simulink model "Incremental_HSMC"  (R2023b)
settings: Solver=ode1  StartTime=0.0  StopTime=60  FixedStep=0.01  RelTol=1e-3
libraries: simulink x1
settings Model: Creator=vanch  LastModifiedBy=vanch

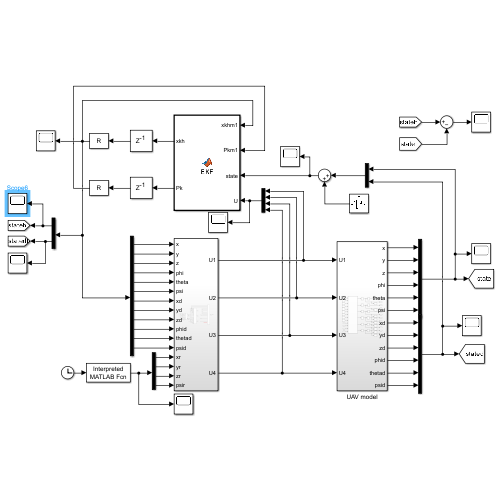
[thumbnail: Simulink's stored preview of the top-level diagram]
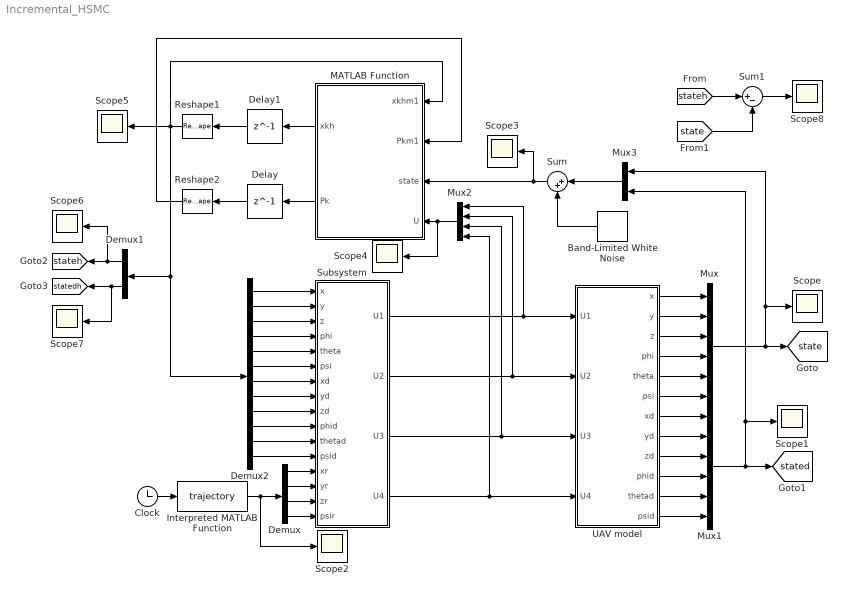
== system Incremental_HSMC ==
  Band-Limited White Noise : simulink/Sources/Band-Limited White Noise  Cov=1e-8  Ts=0.01  seed=[1535]
  Clock : Clock
  Delay : Delay  DelayLength=1  InitialCondition=(1e-3)*eye(12,12)
  Delay1 : Delay  DelayLength=1  InitialCondition=0.001
  Demux : Demux
  Demux1 : Demux  Outputs=2
  Demux2 : Demux  Outputs=12
  Interpreted MATLAB Function : MATLABFcn  MATLABFcn=trajectory  OutputDimensions=4
  MATLAB Function : MATLAB Function  TreatAsAtomicUnit=on
  Mux : Mux  Inputs=6
  Mux1 : Mux  Inputs=6
  Mux2 : Mux
  Mux3 : Mux  Inputs=2
  Reshape1 : Reshape  OutputDimensionality=Customize  OutputDimensions=[12,1]
  Reshape2 : Reshape  OutputDimensionality=Customize  OutputDimensions=[12,12]
  Scope{,1..8} (9 alike) : Scope
  Subsystem : Subsystem
  Sum : Sum  Inputs=|++
  Sum1 : Sum  Inputs=|+-
  UAV model : Subsystem
  tag scope: state=global, stated=global, statedh=global, stateh=global
  wires:
  UAV model/1(x) -> Mux/1
  UAV model/2(y) -> Mux/2
  UAV model/3(z) -> Mux/3
  UAV model/4(phi) -> Mux/4
  UAV model/5(theta) -> Mux/5
  UAV model/6(psi) -> Mux/6
  UAV model/7(xd) -> Mux1/1
  UAV model/8(yd) -> Mux1/2
  UAV model/9(zd) -> Mux1/3
  UAV model/10(phid) -> Mux1/4
  UAV model/11(thetad) -> Mux1/5
  UAV model/12(psid) -> Mux1/6
  Subsystem/3(U3) -> UAV model/3(U3), Mux2/3
  Subsystem/1(U1) -> Mux2/1, UAV model/1(U1)
  Mux/1 -> [state], Scope/1, Mux3/1
  Subsystem/4(U4) -> Mux2/4, UAV model/4(U4)
  Mux3/1 -> Sum/1
  Mux1/1 -> Mux3/2, Scope1/1, [stated]
  Subsystem/2(U2) -> Mux2/2, UAV model/2(U2)
  Mux2/1 -> Scope4/1, MATLAB Function/4(U)
  MATLAB Function/1(xkh) -> Delay1/1
  MATLAB Function/2(Pk) -> Delay/1
  Delay/1 -> Reshape2/1
  Reshape2/1 -> MATLAB Function/2(Pkm1)
  Sum/1 -> MATLAB Function/3(state), Scope3/1
  Delay1/1 -> Reshape1/1
  Demux2/4 -> Subsystem/4(phi)
  Demux2/5 -> Subsystem/5(theta)
  Demux2/6 -> Subsystem/6(psi)
  Demux2/7 -> Subsystem/7(xd)
  Demux2/8 -> Subsystem/8(yd)
  Demux2/9 -> Subsystem/9(zd)
  Demux2/10 -> Subsystem/10(phid)
  Demux2/11 -> Subsystem/11(thetad)
  Demux2/12 -> Subsystem/12(psid)
  Demux2/1 -> Subsystem/1(x)
  Demux2/2 -> Subsystem/2(y)
  Demux2/3 -> Subsystem/3(z)
  Clock/1 -> Interpreted MATLAB Function/1
  Demux/2 -> Subsystem/14(yr)
  Demux/4 -> Subsystem/16(psir)
  Demux/3 -> Subsystem/15(zr)
  Demux/1 -> Subsystem/13(xr)
  Interpreted MATLAB Function/1 -> Demux/1, Scope2/1
  Demux1/2 -> Scope7/1, [statedh]
  Reshape1/1 -> MATLAB Function/1(xkhm1), Demux2/1, Demux1/1, Scope5/1
  Demux1/1 -> Scope6/1, [stateh]
  Sum1/1 -> Scope8/1
  [stateh] -> Sum1/1
  [state] -> Sum1/2
  Band-Limited White Noise/1 -> Sum/2

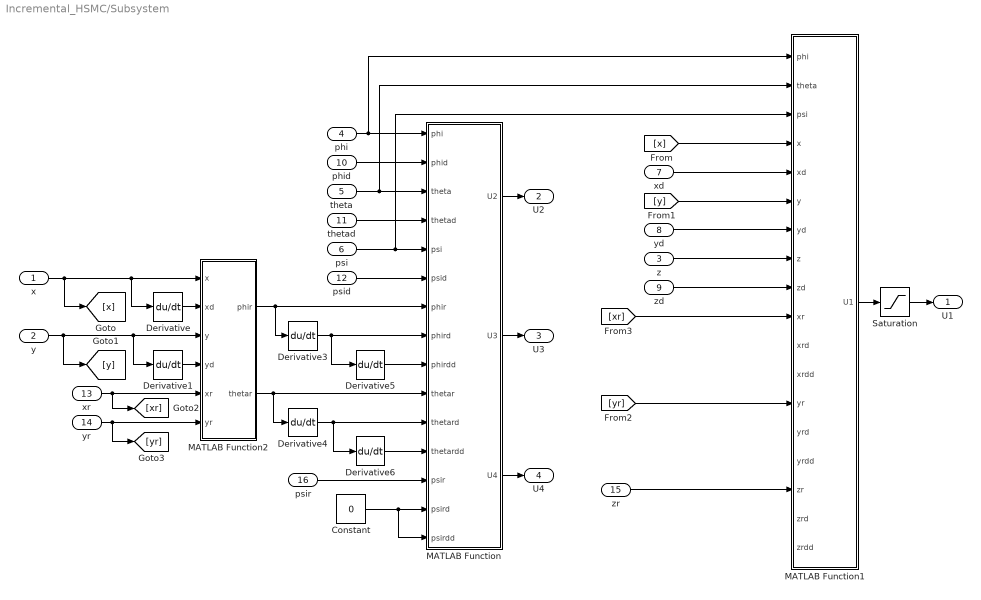
== system Incremental_HSMC/Subsystem ==
  x : Inport
  y : Inport  Port=2
  z : Inport  Port=3
  phi : Inport  Port=4
  theta : Inport  Port=5
  psi : Inport  Port=6
  xd : Inport  Port=7
  yd : Inport  Port=8
  zd : Inport  Port=9
  phid : Inport  Port=10
  thetad : Inport  Port=11
  psid : Inport  Port=12
  xr : Inport  Port=13
  yr : Inport  Port=14
  zr : Inport  Port=15
  psir : Inport  Port=16
  Constant : Constant  Value=0
  Derivative{,1,3..6} (6 alike) : Derivative
  MATLAB Function : MATLAB Function  TreatAsAtomicUnit=on
  MATLAB Function1 : MATLAB Function  TreatAsAtomicUnit=on
  MATLAB Function2 : MATLAB Function  TreatAsAtomicUnit=on
  Saturation : Saturate  UpperLimit=50  LowerLimit=0
  U1 : Outport
  U2 : Outport  Port=2
  U3 : Outport  Port=3
  U4 : Outport  Port=4
  wires:
  x/1 -> Derivative/1, MATLAB Function2/1(x), [x]
  Derivative/1 -> MATLAB Function2/2(xd)
  Derivative1/1 -> MATLAB Function2/4(yd)
  y/1 -> [y], Derivative1/1, MATLAB Function2/3(y)
  xr/1 -> [xr], MATLAB Function2/5(xr)
  yr/1 -> [yr], MATLAB Function2/6(yr)
  MATLAB Function/1(U2) -> U2/1
  MATLAB Function/2(U3) -> U3/1
  MATLAB Function/3(U4) -> U4/1
  phi/1 -> MATLAB Function/1(phi), MATLAB Function1/1(phi)
  theta/1 -> MATLAB Function/3(theta), MATLAB Function1/2(theta)
  psi/1 -> MATLAB Function/5(psi), MATLAB Function1/3(psi)
  MATLAB Function2/1(phir) -> MATLAB Function/7(phir), Derivative3/1
  MATLAB Function2/2(thetar) -> MATLAB Function/10(thetar), Derivative4/1
  phid/1 -> MATLAB Function/2(phid)
  thetad/1 -> MATLAB Function/4(thetad)
  Derivative3/1 -> Derivative5/1, MATLAB Function/8(phird)
  Derivative4/1 -> Derivative6/1, MATLAB Function/11(thetard)
  psid/1 -> MATLAB Function/6(psid)
  psir/1 -> MATLAB Function/13(psir)
  Derivative5/1 -> MATLAB Function/9(phirdd)
  Derivative6/1 -> MATLAB Function/12(thetardd)
  [x] -> MATLAB Function1/4(x)
  [y] -> MATLAB Function1/6(y)
  xd/1 -> MATLAB Function1/5(xd)
  yd/1 -> MATLAB Function1/7(yd)
  z/1 -> MATLAB Function1/8(z)
  zd/1 -> MATLAB Function1/9(zd)
  zr/1 -> MATLAB Function1/16(zr)
  ? -> MATLAB Function1/17(zrd)
  [yr] -> MATLAB Function1/13(yr)
  [xr] -> MATLAB Function1/10(xr)
  Constant/1 -> MATLAB Function/15(psirdd), MATLAB Function/14(psird)
  MATLAB Function1/1(U1) -> Saturation/1
  Saturation/1 -> U1/1

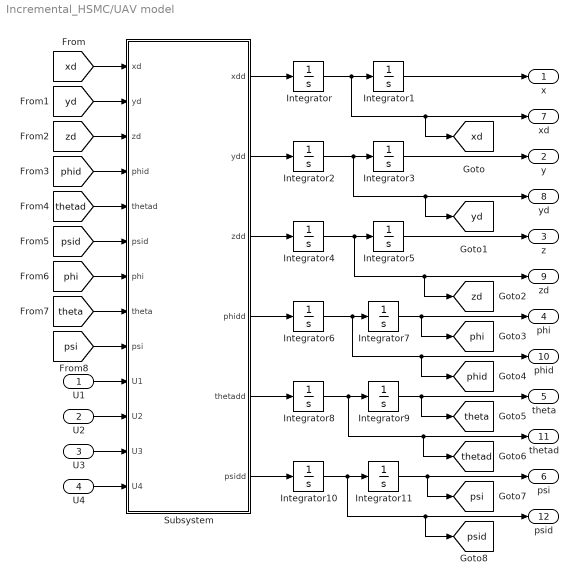
== system Incremental_HSMC/UAV model ==
  U1 : Inport
  U2 : Inport  Port=2
  U3 : Inport  Port=3
  U4 : Inport  Port=4
  Integrator{,1,3,7,9,11} (6 alike) : Integrator  InitialCondition=0.01
  Integrator{2,4,6,8,10} (5 alike) : Integrator
  Integrator5 : Integrator  InitialCondition=0.01  LimitOutput=on  LowerSaturationLimit=0
  Subsystem : Subsystem
  x : Outport
  y : Outport  Port=2
  z : Outport  Port=3
  phi : Outport  Port=4
  theta : Outport  Port=5
  psi : Outport  Port=6
  xd : Outport  Port=7
  yd : Outport  Port=8
  zd : Outport  Port=9
  phid : Outport  Port=10
  thetad : Outport  Port=11
  psid : Outport  Port=12
  tag scope: phi=global, phid=global, psi=global, psid=global, theta=global, thetad=global, xd=global, yd=global, zd=global
  wires:
  Integrator5/1 -> z/1
  Integrator6/1 -> phid/1, [phid], Integrator7/1
  Integrator1/1 -> x/1
  [psid] -> Subsystem/6(psid)
  Integrator2/1 -> yd/1, [yd], Integrator3/1
  Subsystem/3(zdd) -> Integrator4/1
  Subsystem/6(psidd) -> Integrator10/1
  Integrator3/1 -> y/1
  Integrator8/1 -> thetad/1, [thetad], Integrator9/1
  [theta] -> Subsystem/8(theta)
  Integrator/1 -> xd/1, [xd], Integrator1/1
  [thetad] -> Subsystem/5(thetad)
  [zd] -> Subsystem/3(zd)
  Subsystem/4(phidd) -> Integrator6/1
  Integrator9/1 -> theta/1, [theta]
  [phid] -> Subsystem/4(phid)
  Integrator10/1 -> psid/1, [psid], Integrator11/1
  Subsystem/2(ydd) -> Integrator2/1
  Integrator4/1 -> zd/1, [zd], Integrator5/1
  Subsystem/5(thetadd) -> Integrator8/1
  Subsystem/1(xdd) -> Integrator/1
  [yd] -> Subsystem/2(yd)
  [psi] -> Subsystem/9(psi)
  Integrator11/1 -> psi/1, [psi]
  [xd] -> Subsystem/1(xd)
  [phi] -> Subsystem/7(phi)
  Integrator7/1 -> phi/1, [phi]
  U1/1 -> Subsystem/10(U1)
  U2/1 -> Subsystem/11(U2)
  U3/1 -> Subsystem/12(U3)
  U4/1 -> Subsystem/13(U4)

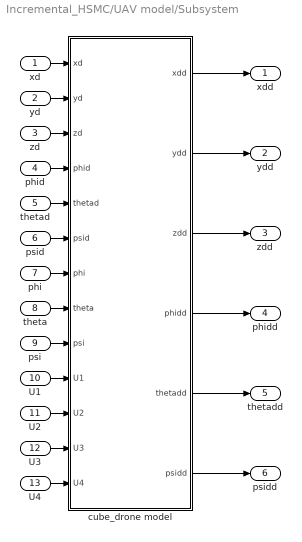
== system Incremental_HSMC/UAV model/Subsystem ==
  xd : Inport
  yd : Inport  Port=2
  zd : Inport  Port=3
  phid : Inport  Port=4
  thetad : Inport  Port=5
  psid : Inport  Port=6
  phi : Inport  Port=7
  theta : Inport  Port=8
  psi : Inport  Port=9
  U1 : Inport  Port=10
  U2 : Inport  Port=11
  U3 : Inport  Port=12
  U4 : Inport  Port=13
  cube_drone model : MATLAB Function  TreatAsAtomicUnit=on
  xdd : Outport
  ydd : Outport  Port=2
  zdd : Outport  Port=3
  phidd : Outport  Port=4
  thetadd : Outport  Port=5
  psidd : Outport  Port=6
  wires:
  U4/1 -> cube_drone model/13(U4)
  U1/1 -> cube_drone model/10(U1)
  U2/1 -> cube_drone model/11(U2)
  cube_drone model/2(ydd) -> ydd/1
  cube_drone model/4(phidd) -> phidd/1
  U3/1 -> cube_drone model/12(U3)
  cube_drone model/3(zdd) -> zdd/1
  cube_drone model/5(thetadd) -> thetadd/1
  psid/1 -> cube_drone model/6(psid)
  cube_drone model/6(psidd) -> psidd/1
  zd/1 -> cube_drone model/3(zd)
  yd/1 -> cube_drone model/2(yd)
  thetad/1 -> cube_drone model/5(thetad)
  phid/1 -> cube_drone model/4(phid)
  phi/1 -> cube_drone model/7(phi)
  cube_drone model/1(xdd) -> xdd/1
  xd/1 -> cube_drone model/1(xd)
  theta/1 -> cube_drone model/8(theta)
  psi/1 -> cube_drone model/9(psi)

== matlab function Incremental_HSMC/MATLAB Function ==
  data: xkhm1 input; Pkm1 input; xkh output; state input; U input; Pk output
function [xkh,Pk] = EKF(xkhm1,Pkm1,state,U)
%parameters
dt=0.01;
Q=1e-5;
R=1e-6;
m=1.96;
g=9.81;
Kdx=0.00055670;
Kdy=0.00055670;
Kdz=0.0006354;
Ixx=0.00149;
Iyy=0.00153;
Izz=0.00532;
%states
x=xkhm1(1);
y=xkhm1(2);
z=xkhm1(3);
phi=xkhm1(4);
theta=xkhm1(5);
psi=xkhm1(6);
xd=xkhm1(7);
yd=xkhm1(8);
zd=xkhm1(9);
phid=xkhm1(10);
thetad=xkhm1(11);
psid=xkhm1(12);
%linearized
A=[0, 0, 0, 0, 0, 0, 1, 0, 0, 0, 0, 0;
   0, 0, 0, 0, 0, 0, 0, 1, 0, 0, 0, 0;
   0, 0, 0, 0, 0, 0, 0, 0, 1, 0, 0, 0;
   0, 0, 0, 0, 0, 0, 0, 0, 0, 1, 0, 0;
   0, 0, 0, 0, 0, 0, 0, 0, 0, 0, 1, 0;
   0, 0, 0, 0, 0, 0, 0, 0, 0, 0, 0, 1;
   0, 0, 0, 0, 0, 0, -Kdx/m, 0, 0, 0, 0, 0;
  0, 0, 0, 0, 0, 0, 0, -Kdy/m, 0, 0, 0, 0;
  0, 0, 0, 0, 0, 0, 0, 0, -Kdz/m, 0, 0, 0;
  0, 0, 0, 0, 0, 0, 0, 0, 0, 0, (psid*(Iyy - Izz))/Ixx, (thetad*(Iyy - Izz))/Ixx;
  0, 0, 0, 0, 0, 0, 0, 0, 0, -(psid*(Ixx - Izz))/Iyy, 0, -(phid*(Ixx - Izz))/Iyy;
  0, 0, 0, 0, 0, 0, 0, 0, 0, (thetad*(Ixx - Iyy))/Izz, (phid*(Ixx - Iyy))/Izz, 0];
B=[0, 0, 0, 0;
   0, 0, 0, 0;
   0, 0, 0, 0;
   0, 0, 0, 0;
   0, 0, 0, 0;
   0, 0, 0, 0;
   (sin(phi)*sin(psi) + cos(phi)*cos(psi)*sin(theta))/m, 0, 0, 0;
   -(cos(psi)*sin(phi) - cos(phi)*sin(psi)*sin(theta))/m, 0, 0, 0;
   (cos(phi)*cos(theta))/m, 0, 0 ,0;
   0, 1/Ixx, 0, 0;
   0, 0, 1/Iyy, 0;
   0, 0, 0, 1/Izz];
%Prediction
xkhm=xkhm1+A*xkhm1*dt+B*U*dt;
Pkm=A*Pkm1*A'+Q*eye(12);
%update
Kk=(Pkm*eye(12))/(eye(12)*Pkm*eye(12)+R*eye(12));
xkh=xkhm+Kk*(state-eye(12)*xkhm);
Pk=(eye(12)-Kk*eye*(12))*Pkm;
end

== matlab function Incremental_HSMC/Subsystem/MATLAB Function ==
  data: phi input; phid input; U2 output; U3 output; U4 output; theta input; thetad input; psi input; psid input; phir input; phird input; phirdd input; thetar input; thetard input; thetardd input; psir input; psird input; psirdd input
function [U2,U3,U4] = fcn(phi,phid,theta,thetad,psi,psid,phir,phird,phirdd,thetar,thetard,thetardd,psir,psird,psirdd)
Ixx=0.00219;
Iyy=0.00432;
Izz=0.00578;
cphi=3.5;
ctheta=3.5;
cpsi=0.5;
fphi=psid*thetad*(Iyy-Izz)/Ixx;
ftheta=psid*phid*(Izz-Ixx)/Iyy;
fpsi=phid*thetad*(Ixx-Iyy)/Izz;
bphi=1/Ixx;
btheta=1/Iyy;
bpsi=1/Izz;
Kphi=0.4;
Ktheta=0.4;
Kpsi=0.2;
sphi=cphi*(phi-phir)+(phid-phird);
stheta=ctheta*(theta-thetar)+(thetad-thetard);
spsi=cpsi*(psi-psir)+(psid-psird);
satphi= min(max(sphi, -1), 1);
sattheta= min(max(stheta, -1), 1);
satpsi= min(max(spsi, -1), 1);

U2=(-cphi*phi-(cphi+1)*phid+cphi*phir+(cphi+1)*phird-fphi-Kphi*satphi)/bphi;
U3=(-ctheta*theta-(ctheta+1)*thetad+ctheta*thetar+(ctheta+1)*thetard-ftheta-Ktheta*sattheta)/btheta;
U4=(-cpsi*psi-(cpsi+1)*psid+cpsi*psir+(cpsi+1)*psird-fpsi-Kpsi*satpsi)/bpsi;

end

== matlab function Incremental_HSMC/UAV model/Subsystem/cube_drone model ==
  data: xd input; xdd output; yd input; zd input; phid input; thetad input; psid input; phi input; theta input; psi input; U1 input; U2 input; U3 input; U4 input; ydd output; zdd output; phidd output; thetadd output; psidd output
function [xdd,ydd,zdd,phidd,thetadd,psidd] = fcn(xd,yd,zd,phid,thetad,psid,phi,theta,psi,U1,U2,U3,U4)
%cos,sin
cphi=cos(phi);
sphi=sin(phi);
ctheta=cos(theta);
stheta=sin(theta);
cpsi=cos(psi);
spsi=sin(psi);
%parameters
m=1.96;
g=9.81;
Kdx=0.00055670;
Kdy=0.00055670;
Kdz=0.0006354;
Ixx=0.00149;
Iyy=0.00153;
Izz=0.00532;
%motion equation
xdd=1/m*((spsi*sphi+cpsi*stheta*cphi)*U1-Kdx*xd);
ydd=1/m*((spsi*stheta*cphi-cpsi*sphi)*U1-Kdy*yd);
zdd=1/m*(ctheta*cphi*U1-Kdz*zd-m*g);
phidd=1/Ixx*(psid*thetad*(Iyy-Izz)+U2);
thetadd=1/Iyy*(psid*phid*(Izz-Ixx)+U3);
psidd=1/Izz*(phid*thetad*(Ixx-Iyy)+U4);
end

== matlab function Incremental_HSMC/Subsystem/MATLAB Function1 ==
  data: phi input; theta input; psi input; x input; U1 output; xd input; y input; yd input; z input; zd input; xr input; xrd input; xrdd input; yr input; yrd input; yrdd input; zr input; zrd input; zrdd input
function U1 = fcn(phi,theta,psi,x,xd,y,yd,z,zd,xr,xrd,xrdd,yr,yrd,yrdd,zr,zrd,zrdd)
%paramters
m=1.96;
g=9.81;
Kdx=0.00055670;
Kdy=0.00055670;
Kdz=0.0006354;
c1=0.05;
c2=0.05;
c3=0.05;
c4=10.5;
c5=3.25;
K=0.75;
eta=0.25;
%functions
cphi=cos(phi);
sphi=sin(phi);
ctheta=cos(theta);
stheta=sin(theta);
cpsi=cos(psi);
spsi=sin(psi);

fx=-Kdx*xd/m;
fy=-Kdy*yd/m;
fz=(-Kdz*zd-m*g)/m;
bx=1/m*(spsi*sphi+cpsi*stheta*cphi);
by=1/m*(spsi*stheta*cphi-cpsi*sphi);
bz=1/m*(ctheta*cphi);

s1=c1*(xd-xrd)+(x-xr);
s2=c2*(y-yr)+s1;
s3=c3*(yd-yrd)+s2;
s4=c4*(z-zr)+s3;
s5=c5*(zd-zrd)+s4;

sats5=min(max(s5, -1), 1);
ueq=-(c5*fz+c3*fy+c1*fx+c4*(zd-zrd)+c2*(yd-yrd)+(xd-xrd)-c5*zrdd-c3*yrdd-c1*xrdd)/(c5*bz+c3*by+c1*bx);
usw=-(K*s5+eta*sats5)/(c5*bz+c3*by+c1*bx);
U1=ueq+usw;
end

== matlab function Incremental_HSMC/Subsystem/MATLAB Function2 ==
  data: x input; phir output; xd input; thetar output; y input; yd input; xr input; yr input
function [phir,thetar] = fcn(x,xd,y,yd,xr,yr)
kpx=0.1;
kdx=0.15;
kpy=0.1;
kdy=0.15;
thetar=kpx*(xr-x)-kdx*xd;
phir=-kpy*(yr-y)+kdy*yd;
end
